simulink model "bike_model"  (R2018a)
settings: Solver=FixedStepAuto  StartTime=0.0  StopTime=10  FixedStep=Ts_IMU  RelTol=1e-3
values from neighbouring files (symbols this model uses):
  A_full = zeros(length(velocity_lqr),3,3)    [bike_init.m]
  A_full_dis = zeros(length(velocity_lqr),3,3)    [bike_init.m]
  amp_dist_roll_rate = 1    [bike_init.m]
  b = 1.095    [bike_init.m]    (also in bike_init_Merged_v1.m = bike3D190215())
  B_full = zeros(length(velocity_lqr),3)    [bike_init.m]
  B_full_dis = zeros(length(velocity_lqr),3)    [bike_init.m]
  C = eye(3)    [bike_init.m]    (also in bike_init_Merged_v1.m)
  complementary = 0.995    [bike_init.m]    (also in bike_init_Merged_v1.m = 0.985)
  cumulative_dist_along_path = [0;cumsum(dist_from_vertex_to_vertex,1)]    [bike_init.m]    (also in bike_init_Merged_v1.m)
  Dead_Band = [0.055,-0.005,0.005]    [bike_init.m]    (also in bike_init_Merged_v1.m = [0.055,-0.055,0.005])
  delay = 0.045    [bike_init.m]    (also in bike_init_Merged_v1.m)
  discrete = 1    [bike_init.m]
  dist_freq = 100    [bike_init.m]
  g = 9.81    [bike_init.m]    (also in bike_init_Merged_v1.m)
  IMU_height = 0.9    [bike_init.m]
  initial_x = x_ini_diff    (= 0)    [bike_init.m]    (also in bike_init_Merged_v1.m)
  initial_y = y_ini_diff    (= 0)    [bike_init.m]    (also in bike_init_Merged_v1.m)
  input_velocity = 2    [bike_init.m]    (also in bike_init_Merged_v1.m = 2.5)
  K_full = zeros(length(velocity_lqr),3)    [bike_init.m]
  K_full_dis = zeros(length(velocity_lqr),3)    [bike_init.m]    (also in bike_init_Merged_v1.m)
  L_full = zeros(length(velocity_lqr),3,3)    [bike_init.m]
  L_full_dis = zeros(length(velocity_lqr),3,3)    [bike_init.m]
  max_handlebar = 40*(pi/180)    (= 0.698131700798)    [bike_init.m]    (also in bike_init_Merged_v1.m)
  max_steering_motor_acc = inf    [bike_init.m]    (also in bike_init_Merged_v1.m)
  max_steering_motor_speed = 7.5    [bike_init.m]    (also in bike_init_Merged_v1.m)
  min_handlebar = -max_handlebar    (= -0.698131700798)    [bike_init.m]    (also in bike_init_Merged_v1.m)
  min_steering_motor_acc = -inf    [bike_init.m]    (also in bike_init_Merged_v1.m)
  min_steering_motor_speed = -7.5    [bike_init.m]    (also in bike_init_Merged_v1.m)
  noise_acc = 0.006*(pi/180)    (= 0.00010471975512)    [bike_init.m]    (also in bike_init_Merged_v1.m)
  noise_encoder = 1e-7    (= 1e-07)    [bike_init.m]    (also in bike_init_Merged_v1.m)
  noise_gyro = 0.001929307*(pi/180)    (= 3.36727594318e-05)    [bike_init.m]    (also in bike_init_Merged_v1.m)
  noise_hall = 0    [bike_init.m]    (also in bike_init_Merged_v1.m)
  parameters = [g h b a]    [bike_init.m]
  path_x = time_array    [bike_init.m]    (also in bike_init_Merged_v1.m)
  path_y = sqrt(path_x * 0.8) .* sin(0.1*path_x)    [bike_init.m]    (also in bike_init_Merged_v1.m)
  roll_rate_coef = 0.8    [bike_init.m]    (also in bike_init_Merged_v1.m = 0.9)
  Ts = 0.04    [bike_init.m]    (also in bike_init_Merged_v1.m)
  Ts_IMU = 0.01    [bike_init.m]    (also in bike_init_Merged_v1.m = 0.04)
  velocity_lqr = linspace(0.001,10,100)    [bike_init.m]    (also in bike_init_Merged_v1.m = [velocity_lqr-0.1 velocity_lqr velocity_lqr+0.1])
undefined symbols (not defined in the file or in its folder): curvature
libraries: simulink x14, dspsigops x2, dspsigattribs x1
(part 1 of 3)
settings Model: Creator=Boaz Ash  LastModifiedBy=Umur

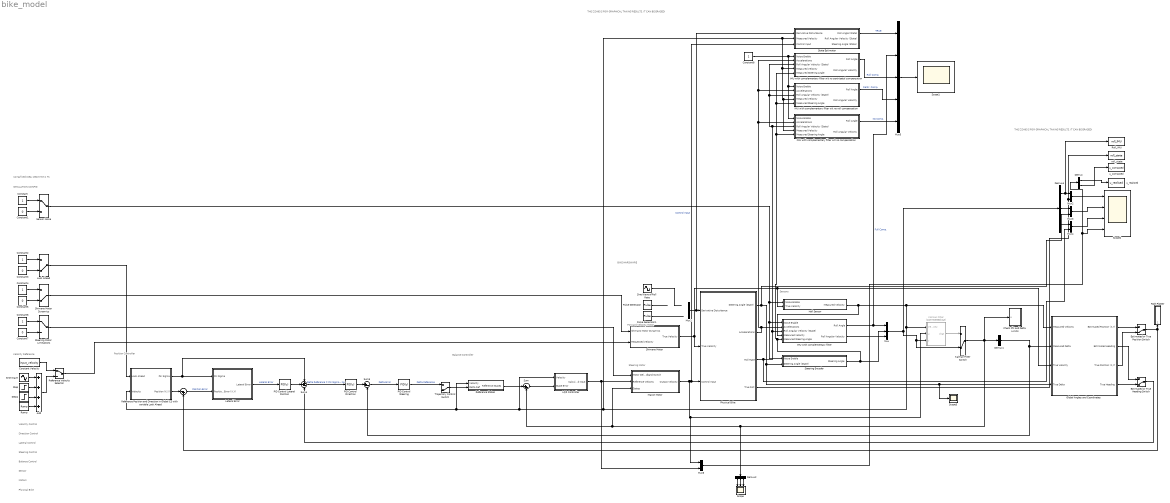
== system bike_model ==
  note: Using fixed step, step time = Ts
  note: SIMULATION CONFIG
  note: BIKE HARDWARE
  note: Direction Control
  note: Steering Control
  note: Lateral Control
  note: Velocity Control
  note: Sensor
  note: Velocity Reference
  note: Sensors
  note: Steering Motor
  note: Balance Control
  note: Forward Velocity Motor
  note: Position Controller
  note: Balance Controller
  note: Motors
  note: Physical Bike
  note: THIS ZONE IS FOR GRAPHICAL TAKING RESULTS. IT CAN BE ERASED!
  note: THIS ZONE IS FOR GRAPHICAL TAKING RESULTS. IT CAN BE ERASED!
  " " : Sum  Inputs=|-+
  Add : Sum  Inputs=4
  Check Phi and Delta Limits : Subsystem  TreatAsAtomicUnit=on  SystemSampleTime=Ts
  Constant{,2,4,6,8} (5 alike) : Constant
  Constant Velocity : Constant  Value=input_velocity
  Constant{1,3,5,7} (4 alike) : Constant  Value=0
  Demux : Demux  Outputs=2
  Demux1 : Demux  Outputs=3
  Demux2 : Demux  Outputs=3
  Demux4 : Demux  Outputs=3
  Estimated or True Heading Switch : ManualSwitch  CurrentSetting=0
  Estimated or True Position Switch : ManualSwitch  CurrentSetting=0
  Global Angles and Coordinates : Subsystem  SystemSampleTime=Ts
  Hall Sensor : Subsystem  TreatAsAtomicUnit=on  SystemSampleTime=Ts
  IMU with complementary filter : Subsystem  SystemSampleTime=Ts_IMU
  IMU with complementary filter wit no centripetal compensation : Subsystem  SystemSampleTime=Ts_IMU
  IMU with complementary filter wit no compensation : Subsystem  SystemSampleTime=Ts_IMU
  IMU with complementary filter wit no roll compensation : Subsystem  SystemSampleTime=Ts_IMU
  Kalman Filter : Subsystem  Commented=on  SystemSampleTime=Ts
  Kalman Filter Switch : ManualSwitch  CurrentSetting=0
  LQR Controller : Subsystem  TreatAsAtomicUnit=on  SystemSampleTime=Ts
  Lateral Error : Subsystem  SystemSampleTime=Ts
  Look Ahead : ManualSwitch  CurrentSetting=0
  Maxon Motor : Subsystem
  Mux : Mux  Inputs=3
  Mux1 : Mux  Inputs=3
  Mux{2..4,6} (4 alike) : Mux  Inputs=2
  Mux5 : Mux  Inputs=5
  PID Control Lateral Position : simulink/Continuous/PID Controller  Controller=PID  TimeDomain=Discrete-time  SampleTime=Ts  IntegratorMethod=Forward Euler  FilterMethod=Forward Euler  Form=Parallel  UseFilter=on  ControllerParametersSource=internal  P=.1  I=.01  D=0  N=100  InitialConditionSource=internal  InitialConditionForIntegrator=0  InitialConditionForFilter=0  ExternalReset=none  LimitOutput=off  UpperSaturationLimit=inf  LowerSaturationLimit=-inf  LinearizeAsGain=on  AntiWindupMode=none  Kb=1  TrackingMode=off  Kt=1  PParamMin=[]  PParamMax=[]  IParamMin=[]  IParamMax=[]  DParamMin=[]  DParamMax=[]  NParamMin=[]  NParamMax=[]  KbParamMin=[]  KbParamMax=[]  KtParamMin=[]  KtParamMax=[]  POutMin=[]  POutMax=[]  IOutMin=[]  IOutMax=[]  DOutMin=[]  DOutMax=[]  NOutMin=[]  NOutMax=[]  KbOutMin=[]  KbOutMax=[]  KtOutMin=[]  KtOutMax=[]  IntegratorOutMin=[]  IntegratorOutMax=[]  FilterOutMin=[]  FilterOutMax=[]  SumOutMin=[]  SumOutMax=[]  SumI1OutMin=[]  SumI1OutMax=[]  SumI2OutMin=[]  SumI2OutMax=[]  SumI3OutMin=[]  SumI3OutMax=[]  SumDOutMin=[]  SumDOutMax=[]  SaturationOutMin=[]  SaturationOutMax=[]  IntegratorContinuousStateAttributes=''  IntegratorStateMustResolveToSignalObject=off  IntegratorRTWStateStorageClass=Auto  FilterContinuousStateAttributes=''  FilterStateMustResolveToSignalObject=off  FilterRTWStateStorageClass=Auto  DifferentiatorICPrevScaledInput=0  DifferentiatorOutMin=[]  DifferentiatorOutMax=[]  FilterDiffOutCoefMin=[]  FilterDiffOutCoefMax=[]  SumDenOutMin=[]  SumDenOutMax=[]  SumNumOutMin=[]  SumNumOutMax=[]  ReciprocalOutMin=[]  ReciprocalOutMax=[]  DivideOutMin=[]  DivideOutMax=[]  TunerSelectOption=Transfer Function Based (PID Tuner App)
  PID Control Direction : simulink/Continuous/PID Controller  Controller=PID  TimeDomain=Discrete-time  SampleTime=Ts  IntegratorMethod=Forward Euler  FilterMethod=Forward Euler  Form=Parallel  UseFilter=on  ControllerParametersSource=internal  P=0.8  I=0.4  D=0  N=100  InitialConditionSource=internal  InitialConditionForIntegrator=0  InitialConditionForFilter=0  ExternalReset=none  LimitOutput=off  UpperSaturationLimit=inf  LowerSaturationLimit=-inf  LinearizeAsGain=on  AntiWindupMode=none  Kb=1  TrackingMode=off  Kt=1  PParamMin=[]  PParamMax=[]  IParamMin=[]  IParamMax=[]  DParamMin=[]  DParamMax=[]  NParamMin=[]  NParamMax=[]  KbParamMin=[]  KbParamMax=[]  KtParamMin=[]  KtParamMax=[]  POutMin=[]  POutMax=[]  IOutMin=[]  IOutMax=[]  DOutMin=[]  DOutMax=[]  NOutMin=[]  NOutMax=[]  KbOutMin=[]  KbOutMax=[]  KtOutMin=[]  KtOutMax=[]  IntegratorOutMin=[]  IntegratorOutMax=[]  FilterOutMin=[]  FilterOutMax=[]  SumOutMin=[]  SumOutMax=[]  SumI1OutMin=[]  SumI1OutMax=[]  SumI2OutMin=[]  SumI2OutMax=[]  SumI3OutMin=[]  SumI3OutMax=[]  SumDOutMin=[]  SumDOutMax=[]  SaturationOutMin=[]  SaturationOutMax=[]  IntegratorContinuousStateAttributes=''  IntegratorStateMustResolveToSignalObject=off  IntegratorRTWStateStorageClass=Auto  FilterContinuousStateAttributes=''  FilterStateMustResolveToSignalObject=off  FilterRTWStateStorageClass=Auto  DifferentiatorICPrevScaledInput=0  DifferentiatorOutMin=[]  DifferentiatorOutMax=[]  FilterDiffOutCoefMin=[]  FilterDiffOutCoefMax=[]  SumDenOutMin=[]  SumDenOutMax=[]  SumNumOutMin=[]  SumNumOutMax=[]  ReciprocalOutMin=[]  ReciprocalOutMax=[]  DivideOutMin=[]  DivideOutMax=[]  TunerSelectOption=Transfer Function Based (PID Tuner App)
  PID Control Steering : simulink/Continuous/PID Controller  Controller=PID  TimeDomain=Discrete-time  SampleTime=Ts  IntegratorMethod=Forward Euler  FilterMethod=Forward Euler  Form=Parallel  UseFilter=on  ControllerParametersSource=internal  P=1  I=0.1  D=0  N=100  InitialConditionSource=internal  InitialConditionForIntegrator=0  InitialConditionForFilter=0  ExternalReset=none  LimitOutput=off  UpperSaturationLimit=inf  LowerSaturationLimit=-inf  LinearizeAsGain=on  AntiWindupMode=none  Kb=1  TrackingMode=off  Kt=1  PParamMin=[]  PParamMax=[]  IParamMin=[]  IParamMax=[]  DParamMin=[]  DParamMax=[]  NParamMin=[]  NParamMax=[]  KbParamMin=[]  KbParamMax=[]  KtParamMin=[]  KtParamMax=[]  POutMin=[]  POutMax=[]  IOutMin=[]  IOutMax=[]  DOutMin=[]  DOutMax=[]  NOutMin=[]  NOutMax=[]  KbOutMin=[]  KbOutMax=[]  KtOutMin=[]  KtOutMax=[]  IntegratorOutMin=[]  IntegratorOutMax=[]  FilterOutMin=[]  FilterOutMax=[]  SumOutMin=[]  SumOutMax=[]  SumI1OutMin=[]  SumI1OutMax=[]  SumI2OutMin=[]  SumI2OutMax=[]  SumI3OutMin=[]  SumI3OutMax=[]  SumDOutMin=[]  SumDOutMax=[]  SaturationOutMin=[]  SaturationOutMax=[]  IntegratorContinuousStateAttributes=''  IntegratorStateMustResolveToSignalObject=off  IntegratorRTWStateStorageClass=Auto  FilterContinuousStateAttributes=''  FilterStateMustResolveToSignalObject=off  FilterRTWStateStorageClass=Auto  DifferentiatorICPrevScaledInput=0  DifferentiatorOutMin=[]  DifferentiatorOutMax=[]  FilterDiffOutCoefMin=[]  FilterDiffOutCoefMax=[]  SumDenOutMin=[]  SumDenOutMax=[]  SumNumOutMin=[]  SumNumOutMax=[]  ReciprocalOutMin=[]  ReciprocalOutMax=[]  DivideOutMin=[]  DivideOutMax=[]  TunerSelectOption=Transfer Function Based (PID Tuner App)
  Path Plotter : Subsystem  SystemSampleTime=Ts
  Physical Bike : Subsystem
  Pulse Generator : DiscretePulseGenerator  PulseType=Time based  Amplitude=pi/36  Period=100  PhaseDelay=0.1
  Pulse Generator1 : DiscretePulseGenerator  PulseType=Time based  Amplitude=0.5*1.1*(20*pi)/36  Period=100  PhaseDelay=1
  Ramp : simulink/Sources/Ramp  slope=0.03  start=0  InitialOutput=0
  Reference Velocity Selector : ManualSwitch
  Reference Position and Direction in Global CS with variable Look Ahead : Subsystem
  Reference States : Subsystem  SystemSampleTime=Ts
  Roll_IMU : ToWorkspace  VariableName=roll_IMU  SaveFormat=Timeseries  SampleTime=-1
  Scope : Scope  NumInputPorts=3
  Scope1 : Scope
  Scope2 : Scope  NumInputPorts=4
  Scope3 : Scope
  Sensor Noise : ManualSwitch
  Shimano Motor : Subsystem
  Shimano Motor Dynamics : ManualSwitch  CurrentSetting=0
  Sine Wave : Sin  Amplitude=0  SampleTime=0
  Sine Wave of Roll Rate : Sin  Amplitude=amp_dist_roll_rate  Frequency=dist_freq  SampleTime=0
  State Estimator : Subsystem
  Steering Encoder : Subsystem  TreatAsAtomicUnit=on  SystemSampleTime=Ts
  Steering Motor Limitations : ManualSwitch
  Step : Step  Time=20  Before=4  After=8  SampleTime=0
  Step1 : Step  Time=40  After=-1  SampleTime=0
  Sum : Sum  Inputs=|+-
  Sum4 : Sum  Inputs=+--
  Sum5 : Sum  Inputs=|+-
  Trajectory Control Switch : ManualSwitch  CurrentSetting=0
  roll_state : ToWorkspace  VariableName=roll_state  SaveFormat=Timeseries  SampleTime=-1
  u_computed : ToWorkspace  VariableName=u_computed  SaveFormat=Timeseries  SampleTime=-1
  u_realised : ToWorkspace  VariableName=u_realised  SaveFormat=Timeseries  SampleTime=-1
  wires:
  Ramp/1 -> Add/4
  Step/1 -> Add/2
  Add/1 -> Reference Velocity Selector/2
  Sine Wave/1 -> Add/1
  Constant Velocity/1 -> Reference Velocity Selector/1
  Step1/1 -> Add/3
  " "/1 -> Lateral Error/2(Position Error (X,Y))  "Position Error"
  Estimated or True Position Switch/1 -> " "/2, Path Plotter/1(Position)
  Lateral Error/1(Lateral Error) -> PID Control Lateral Position/1  "Lateral Error"
  PID Control Steering/1 -> Trajectory Control Switch/1  "Delta Reference"
  Sum5/1 -> PID Control Steering/1  "Delta Error"
  PID Control Direction/1 -> Sum5/1
  Sum4/1 -> PID Control Direction/1  "Delta Reference = Psi Sigma - Nu"
  Reference Position and Direction in Global CS with variable Look Ahead/2(Position (X,Y)) -> " "/1
  Reference Position and Direction in Global CS with variable Look Ahead/1(Psi Sigma) -> Lateral Error/1(Psi Sigma), Sum4/1
  Estimated or True Heading Switch/1 -> Sum4/3
  Maxon Motor/1(Output Velocity) -> State Estimator/3(Control Input), Physical Bike/3(Control Input), Mux6/1, Kalman Filter/2(u)  "Control Input"
  Sum/1 -> LQR Controller/2(State Error)
  Kalman Filter Switch/1 -> Check Phi and Delta Limits/1(x), Sum/2, Maxon Motor/3(States), Demux2/1, Demux1/1
  Constant/1 -> Sensor Noise/1
  Constant1/1 -> Sensor Noise/2
  Sensor Noise/1 -> Hall Sensor/1(Noise Enable), Steering Encoder/1(Noise Enable), IMU with complementary filter/1(Noise Enable)
  IMU with complementary filter/1(Roll Angle) -> Mux/1, Mux5/2  "Full Comp."
  IMU with complementary filter/2(Roll Angular Velocity) -> Mux/3
  Mux1/1 -> State Estimator/1(Derivative Disturbance), Physical Bike/1(Derivative Disturbance)
  Reference States/1(Reference States) -> Sum/1
  Demux1/2 -> Sum5/2, Global Angles and Coordinates/2(Measured Delta)
  Constant3/1 -> Look Ahead/2
  Constant2/1 -> Look Ahead/1
  Look Ahead/1 -> Reference Position and Direction in Global CS with variable Look Ahead/1(Look Ahead)
  Constant4/1 -> Shimano Motor Dynamics/1
  Constant5/1 -> Shimano Motor Dynamics/2
  Global Angles and Coordinates/1(Estimated Position (X,Y)) -> Estimated or True Position Switch/1
  Global Angles and Coordinates/3(True Position (X,Y)) -> Estimated or True Position Switch/2
  Global Angles and Coordinates/2(Estimated Heading) -> Estimated or True Heading Switch/1
  Global Angles and Coordinates/4(True Heading) -> Estimated or True Heading Switch/2
  Reference Velocity Selector/1 -> Shimano Motor/2(Requested Velocity)
  Demux2/1 -> Scope/1
  Demux2/2 -> Scope/2
  Demux2/3 -> Scope/3
  Steering Motor Limitations/1 -> Maxon Motor/1(Motor Delay & Deadband Switch)
  Constant6/1 -> Steering Motor Limitations/1
  Constant7/1 -> Steering Motor Limitations/2
  Mux/1 -> Kalman Filter/3(y), Kalman Filter Switch/2, Demux4/1
  Kalman Filter/1(xhat) -> Kalman Filter Switch/1
  Shimano Motor/1(True Velocity) -> Hall Sensor/2(True Velocity), Global Angles and Coordinates/3(True Velocity), Physical Bike/2(True Velocity)
  Pulse Generator/1 -> ?
  Shimano Motor Dynamics/1 -> Shimano Motor/1(Shimano Motor Dynamics)
  PID Control Lateral Position/1 -> Sum4/2
  Mux2/1 -> Scope2/1
  Mux3/1 -> Scope2/2
  Mux4/1 -> Scope2/3
  Physical Bike/4(True Roll) -> Mux2/2, roll_state/1
  Physical Bike/1(Steering Angle (State)) -> Mux3/2, Steering Encoder/2(Steering Angle (State)), Scope3/1, Global Angles and Coordinates/4(True Delta)
  Demux4/2 -> Mux3/1
  Demux4/3 -> Mux4/1
  Physical Bike/3(Roll Rate) -> Mux4/2, IMU with complementary filter/3(Roll Angular Velocity (State)), IMU with complementary filter wit no centripetal compensation/3(Roll Angular Velocity (State)), IMU with complementary filter wit no roll compensation/3(Roll Angular Velocity (State)), IMU with complementary filter wit no compensation/3(Roll Angular Velocity (State))
  Trajectory Control Switch/1 -> Reference States/2(Delta Ref)
  Pulse Generator1/1 -> ?
  State Estimator/1(Roll Angle (State)) -> Mux5/1  "TRUE"
  Steering Encoder/1(Steering Angle) -> Mux/2, IMU with complementary filter/5(Measured Steering Angle), IMU with complementary filter wit no compensation/5(Measured Steering Angle), IMU with complementary filter wit no roll compensation/5(Measured Steering Angle), IMU with complementary filter wit no centripetal compensation/5(Measured Steering Angle)
  Mux5/1 -> Scope1/1
  Hall Sensor/1(Measured Velocity) -> IMU with complementary filter/4(Measured Velocity), Kalman Filter/1(Velocity), LQR Controller/1(Velocity), Reference States/1(Velocity), Reference Position and Direction in Global CS with variable Look Ahead/2(Velocity), IMU with complementary filter wit no compensation/4(Measured Velocity), IMU with complementary filter wit no roll compensation/4(Measured Velocity), IMU with complementary filter wit no centripetal compensation/4(Measured Velocity), State Estimator/2(Measured Velocity), Global Angles and Coordinates/1(Measured Velocity)
  Physical Bike/2(Accelerations) -> IMU with complementary filter/2(Accelerations), IMU with complementary filter wit no centripetal compensation/2(Accelerations), IMU with complementary filter wit no roll compensation/2(Accelerations), IMU with complementary filter wit no compensation/2(Accelerations)
  Constant8/1 -> IMU with complementary filter wit no compensation/1(Noise Enable), IMU with complementary filter wit no roll compensation/1(Noise Enable), IMU with complementary filter wit no centripetal compensation/1(Noise Enable)
  IMU with complementary filter wit no centripetal compensation/1(Roll Angle) -> Mux5/3  "Roll Comp."
  IMU with complementary filter wit no roll compensation/1(Roll Angle) -> Mux5/4  "Centr. Comp."
  IMU with complementary filter wit no compensation/1(Roll Angle) -> Mux5/5  "No Comp."
  Sine Wave of Roll Rate/1 -> ?
  LQR Controller/1(Calculated Input) -> Mux6/2, Maxon Motor/2(Reference Velocity)
  Mux6/1 -> Scope2/4, Demux/1
  Demux4/1 -> Roll_IMU/1, Mux2/1
  Demux/2 -> u_computed/1
  Demux/1 -> u_realised/1

== system bike_model/Check Phi and Delta Limits ==
  x : Inport
  Demux : Demux  Outputs=3
  Handlebar Lower Bound : simulink/Model Verification/Check Static  Lower Bound  Description=min_handlebar <= u  min=min_handlebar  min_included=on  enabled=on  stopWhenAssertionFail=on  export=on  icon=graphic
      settings: SourceProductName=Simulink
  Handlebar Upper Bound : simulink/Model Verification/Check Static  Upper Bound  Description=u <= max_handlebar  max=max_handlebar  max_included=on  enabled=on  stopWhenAssertionFail=on  export=on  icon=graphic
      settings: SourceProductName=Simulink  SourceProductBaseCode=SL
  Roll Lower Bound : simulink/Model Verification/Check Static  Lower Bound  Description=min_roll <= u  min=min_roll  min_included=on  enabled=on  stopWhenAssertionFail=on  export=on  icon=graphic
      settings: SourceProductName=Simulink
  Roll Upper Bound : simulink/Model Verification/Check Static  Upper Bound  Description=u <= max_roll  max=max_roll  max_included=on  enabled=on  stopWhenAssertionFail=on  export=on  icon=graphic
      settings: SourceProductName=Simulink  SourceProductBaseCode=SL
  wires:
  Demux/1 -> Roll Lower Bound/1, Roll Upper Bound/1  "Roll Angle"
  ? -> Handlebar Upper Bound/1, Handlebar Lower Bound/1  "Handlebar Angle"
  x/1 -> Demux/1

== system bike_model/Global Angles and Coordinates ==
  Measured Velocity : Inport
  Measured Delta : Inport  Port=2
  True Velocity : Inport  Port=3
  True Delta : Inport  Port=4
  Measured Bike Angles to Global Angles : Subsystem
  Measured Global Angles to Global Coordinates : Subsystem
  Sum : Sum  Inputs=++|
  Sum1 : Sum  Inputs=++|
  True Bike Angles to Global Angles2 : Subsystem
  True Global Angles to Global Coordinates : Subsystem
  Estimated Position (X,Y) : Outport
  Estimated Heading : Outport  Port=2
  True Position (X,Y) : Outport  Port=3
  True Heading : Outport  Port=4
  wires:
  Measured Global Angles to Global Coordinates/1("Position (X, Y)") -> Estimated Position (X,Y)/1
  Measured Velocity/1 -> Measured Global Angles to Global Coordinates/1(Velocity), Measured Bike Angles to Global Angles/1(Velocity)
  Measured Bike Angles to Global Angles/1(psi) -> Sum/2, Measured Global Angles to Global Coordinates/2(Psi)
  True Global Angles to Global Coordinates/1("Position (X, Y)") -> True Position (X,Y)/1
  True Delta/1 -> True Bike Angles to Global Angles2/2(Steering Angle)
  True Velocity/1 -> True Global Angles to Global Coordinates/1(Velocity), True Bike Angles to Global Angles2/1(Velocity)
  Measured Bike Angles to Global Angles/2(beta) -> Measured Global Angles to Global Coordinates/3(Beta), Sum/1
  Measured Delta/1 -> Measured Bike Angles to Global Angles/2(Steering Angle)
  Sum/1 -> Estimated Heading/1
  Sum1/1 -> True Heading/1
  True Bike Angles to Global Angles2/1(psi) -> Sum1/2, True Global Angles to Global Coordinates/2(Psi)
  True Bike Angles to Global Angles2/2(beta) -> Sum1/1, True Global Angles to Global Coordinates/3(Beta)

== system bike_model/Hall Sensor ==
  Noise Enable : Inport
  True Velocity : Inport  Port=2
  Noise on hall sensor : RandomNumber  Variance=noise_hall  Seed=1  SampleTime=Ts
  Saturate Signal : Switch  Criteria=u2 > Threshold
  Sum : Sum  Inputs=++|
  Switch : Switch  Criteria=u2 > Threshold
  Velocity Lower Bound : simulink/Model Verification/Check Static  Lower Bound  Description=0.6 <= u  min=0.6  min_included=on  enabled=on  stopWhenAssertionFail=off  export=on  icon=graphic
      settings: SourceProductName=Simulink
  Zero : Constant  Value=0
  Zero-Order Hold : ZeroOrderHold  SampleTime=Ts
  Measured Velocity : Outport
  wires:
  True Velocity/1 -> Sum/2, Switch/3
  Noise Enable/1 -> Switch/2
  Switch/1 -> Saturate Signal/1, Velocity Lower Bound/1
  Noise on hall sensor/1 -> Sum/1
  Sum/1 -> Switch/1
  Zero/1 -> Saturate Signal/3
  Velocity Lower Bound/1 -> Saturate Signal/2
  Saturate Signal/1 -> Zero-Order Hold/1
  Zero-Order Hold/1 -> Measured Velocity/1

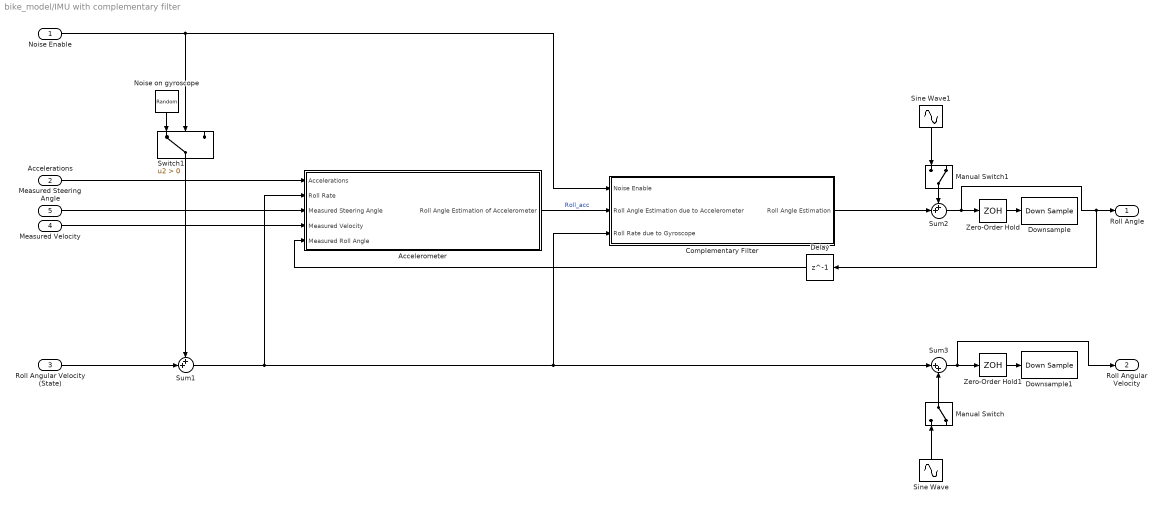
== system bike_model/IMU with complementary filter ==
  Noise Enable : Inport
  Accelerations : Inport  Port=2
  Roll Angular Velocity (State) : Inport  Port=3
  Measured Velocity : Inport  Port=4
  Measured Steering Angle : Inport  Port=5
  Accelerometer : Subsystem
  Complementary Filter : Subsystem  TreatAsAtomicUnit=on  SystemSampleTime=Ts_IMU
  Delay : Delay  DelayLength=1
  Downsample : DownSample  N=Ts/Ts_IMU  RateOptions=Allow multirate processing
  Downsample1 : DownSample  N=Ts/Ts_IMU  RateOptions=Allow multirate processing
  Manual Switch : ManualSwitch  CurrentSetting=0
  Manual Switch1 : ManualSwitch  CurrentSetting=0
  Noise on gyroscope : RandomNumber  Variance=noise_gyro  Seed=1  SampleTime=Ts_IMU
  Sine Wave : Sin  Amplitude=0.05  Frequency=25  SampleTime=Ts_IMU
  Sine Wave1 : Sin  Amplitude=0.02  Frequency=25  Phase=pi  SampleTime=Ts_IMU
  Sum1 : Sum  Inputs=++|
  Sum2 : Sum  Inputs=++|
  Sum3 : Sum  Inputs=|++
  Switch1 : Switch  Criteria=u2 > Threshold
  Zero-Order Hold : ZeroOrderHold  SampleTime=Ts_IMU
  Zero-Order Hold1 : ZeroOrderHold  SampleTime=Ts_IMU
  Roll Angle : Outport
  Roll Angular Velocity : Outport  Port=2
  wires:
  Noise Enable/1 -> Complementary Filter/1(Noise Enable), Switch1/2
  Roll Angular Velocity (State)/1 -> Sum1/2
  Noise on gyroscope/1 -> Switch1/1
  Accelerometer/1(Roll Angle Estimation of Accelerometer) -> Complementary Filter/2(Roll Angle Estimation due to Accelerometer)  "Roll_acc"
  Complementary Filter/1(Roll Angle Estimation) -> Sum2/2
  Switch1/1 -> Sum1/1
  Sine Wave1/1 -> Manual Switch1/1
  Manual Switch1/1 -> Sum2/1
  Sum2/1 -> Delay/1, Roll Angle/1, Zero-Order Hold/1
  Sum3/1 -> Roll Angular Velocity/1, Zero-Order Hold1/1
  Zero-Order Hold/1 -> Downsample/1
  Zero-Order Hold1/1 -> Downsample1/1
  Sum1/1 -> Accelerometer/2(Roll Rate), Complementary Filter/3(Roll Rate due to Gyroscope), Sum3/1
  Sine Wave/1 -> Manual Switch/1
  Manual Switch/1 -> Sum3/2
  Accelerations/1 -> Accelerometer/1(Accelerations)
  Measured Steering Angle/1 -> Accelerometer/3(Measured Steering Angle)
  Measured Velocity/1 -> Accelerometer/4(Measured Velocity)
  Delay/1 -> Accelerometer/5(Measured Roll Angle)

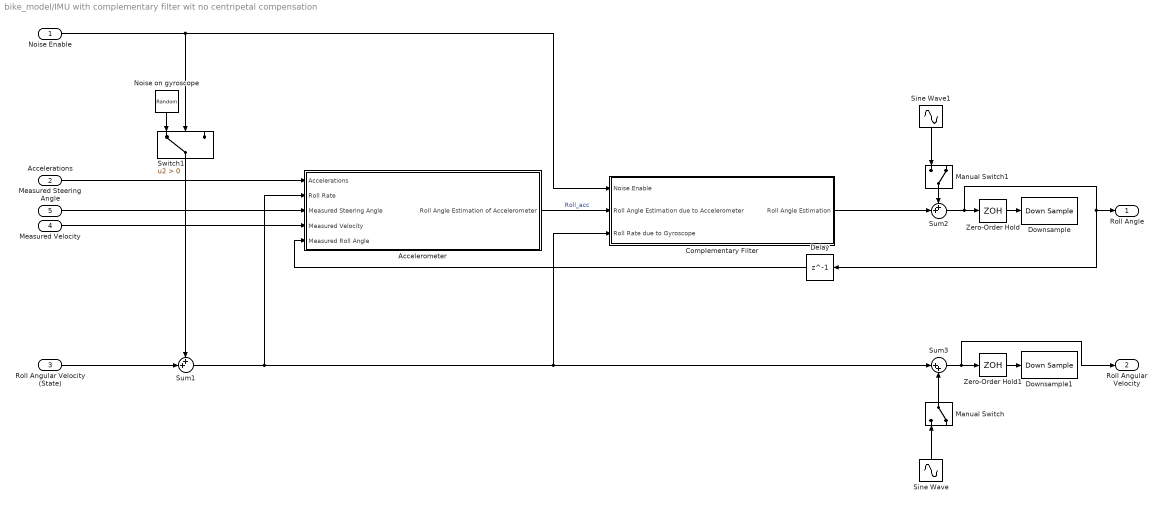
== system bike_model/IMU with complementary filter wit no centripetal compensation ==
  Noise Enable : Inport
  Accelerations : Inport  Port=2
  Roll Angular Velocity (State) : Inport  Port=3
  Measured Velocity : Inport  Port=4
  Measured Steering Angle : Inport  Port=5
  Accelerometer : Subsystem
  Complementary Filter : Subsystem  TreatAsAtomicUnit=on  SystemSampleTime=Ts_IMU
  Delay : Delay  DelayLength=1
  Downsample : DownSample  N=Ts/Ts_IMU  RateOptions=Allow multirate processing
  Downsample1 : DownSample  N=Ts/Ts_IMU  RateOptions=Allow multirate processing
  Manual Switch : ManualSwitch  CurrentSetting=0
  Manual Switch1 : ManualSwitch  CurrentSetting=0
  Noise on gyroscope : RandomNumber  Variance=noise_gyro  Seed=1  SampleTime=Ts_IMU
  Sine Wave : Sin  Amplitude=0.05  Frequency=25  SampleTime=Ts_IMU
  Sine Wave1 : Sin  Amplitude=0.02  Frequency=25  Phase=pi  SampleTime=Ts_IMU
  Sum1 : Sum  Inputs=++|
  Sum2 : Sum  Inputs=++|
  Sum3 : Sum  Inputs=|++
  Switch1 : Switch  Criteria=u2 > Threshold
  Zero-Order Hold : ZeroOrderHold  SampleTime=Ts_IMU
  Zero-Order Hold1 : ZeroOrderHold  SampleTime=Ts_IMU
  Roll Angle : Outport
  Roll Angular Velocity : Outport  Port=2
  wires:
  Noise Enable/1 -> Complementary Filter/1(Noise Enable), Switch1/2
  Roll Angular Velocity (State)/1 -> Sum1/2
  Noise on gyroscope/1 -> Switch1/1
  Accelerometer/1(Roll Angle Estimation of Accelerometer) -> Complementary Filter/2(Roll Angle Estimation due to Accelerometer)  "Roll_acc"
  Complementary Filter/1(Roll Angle Estimation) -> Sum2/2
  Switch1/1 -> Sum1/1
  Sine Wave1/1 -> Manual Switch1/1
  Manual Switch1/1 -> Sum2/1
  Sum2/1 -> Delay/1, Roll Angle/1, Zero-Order Hold/1
  Sum3/1 -> Roll Angular Velocity/1, Zero-Order Hold1/1
  Zero-Order Hold/1 -> Downsample/1
  Zero-Order Hold1/1 -> Downsample1/1
  Sum1/1 -> Accelerometer/2(Roll Rate), Complementary Filter/3(Roll Rate due to Gyroscope), Sum3/1
  Sine Wave/1 -> Manual Switch/1
  Manual Switch/1 -> Sum3/2
  Accelerations/1 -> Accelerometer/1(Accelerations)
  Measured Steering Angle/1 -> Accelerometer/3(Measured Steering Angle)
  Measured Velocity/1 -> Accelerometer/4(Measured Velocity)
  Delay/1 -> Accelerometer/5(Measured Roll Angle)

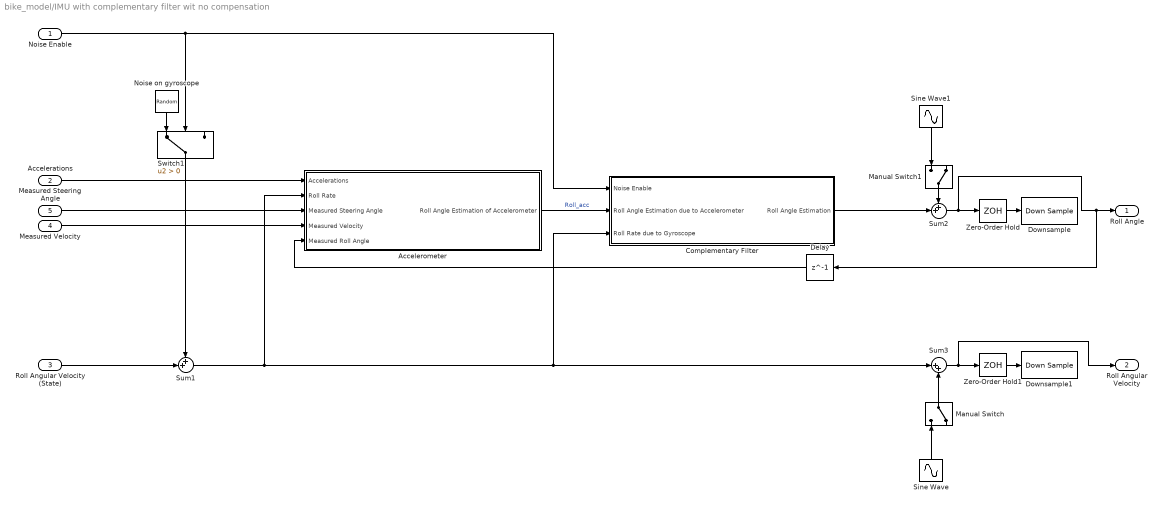
== system bike_model/IMU with complementary filter wit no compensation ==
  Noise Enable : Inport
  Accelerations : Inport  Port=2
  Roll Angular Velocity (State) : Inport  Port=3
  Measured Velocity : Inport  Port=4
  Measured Steering Angle : Inport  Port=5
  Accelerometer : Subsystem
  Complementary Filter : Subsystem  TreatAsAtomicUnit=on  SystemSampleTime=Ts_IMU
  Delay : Delay  DelayLength=1
  Downsample : DownSample  N=Ts/Ts_IMU  RateOptions=Allow multirate processing
  Downsample1 : DownSample  N=Ts/Ts_IMU  RateOptions=Allow multirate processing
  Manual Switch : ManualSwitch  CurrentSetting=0
  Manual Switch1 : ManualSwitch  CurrentSetting=0
  Noise on gyroscope : RandomNumber  Variance=noise_gyro  Seed=1  SampleTime=Ts_IMU
  Sine Wave : Sin  Amplitude=0.05  Frequency=25  SampleTime=Ts_IMU
  Sine Wave1 : Sin  Amplitude=0.02  Frequency=25  Phase=pi  SampleTime=Ts_IMU
  Sum1 : Sum  Inputs=++|
  Sum2 : Sum  Inputs=++|
  Sum3 : Sum  Inputs=|++
  Switch1 : Switch  Criteria=u2 > Threshold
  Zero-Order Hold : ZeroOrderHold  SampleTime=Ts_IMU
  Zero-Order Hold1 : ZeroOrderHold  SampleTime=Ts_IMU
  Roll Angle : Outport
  Roll Angular Velocity : Outport  Port=2
  wires:
  Noise Enable/1 -> Complementary Filter/1(Noise Enable), Switch1/2
  Roll Angular Velocity (State)/1 -> Sum1/2
  Noise on gyroscope/1 -> Switch1/1
  Accelerometer/1(Roll Angle Estimation of Accelerometer) -> Complementary Filter/2(Roll Angle Estimation due to Accelerometer)  "Roll_acc"
  Complementary Filter/1(Roll Angle Estimation) -> Sum2/2
  Switch1/1 -> Sum1/1
  Sine Wave1/1 -> Manual Switch1/1
  Manual Switch1/1 -> Sum2/1
  Sum2/1 -> Delay/1, Roll Angle/1, Zero-Order Hold/1
  Sum3/1 -> Roll Angular Velocity/1, Zero-Order Hold1/1
  Zero-Order Hold/1 -> Downsample/1
  Zero-Order Hold1/1 -> Downsample1/1
  Sum1/1 -> Accelerometer/2(Roll Rate), Complementary Filter/3(Roll Rate due to Gyroscope), Sum3/1
  Sine Wave/1 -> Manual Switch/1
  Manual Switch/1 -> Sum3/2
  Accelerations/1 -> Accelerometer/1(Accelerations)
  Measured Steering Angle/1 -> Accelerometer/3(Measured Steering Angle)
  Measured Velocity/1 -> Accelerometer/4(Measured Velocity)
  Delay/1 -> Accelerometer/5(Measured Roll Angle)

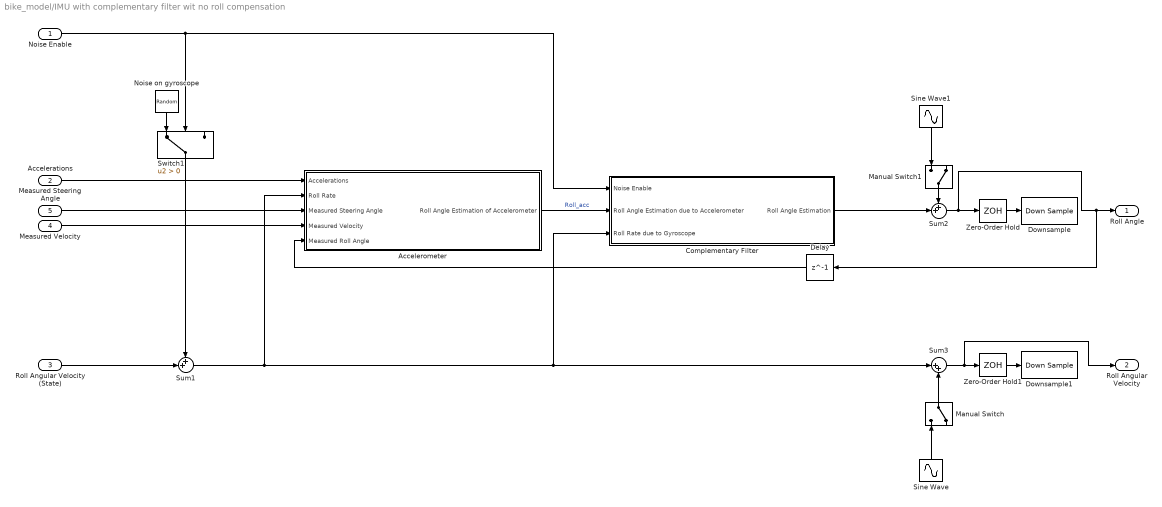
== system bike_model/IMU with complementary filter wit no roll compensation ==
  Noise Enable : Inport
  Accelerations : Inport  Port=2
  Roll Angular Velocity (State) : Inport  Port=3
  Measured Velocity : Inport  Port=4
  Measured Steering Angle : Inport  Port=5
  Accelerometer : Subsystem
  Complementary Filter : Subsystem  TreatAsAtomicUnit=on  SystemSampleTime=Ts_IMU
  Delay : Delay  DelayLength=1
  Downsample : DownSample  N=Ts/Ts_IMU  RateOptions=Allow multirate processing
  Downsample1 : DownSample  N=Ts/Ts_IMU  RateOptions=Allow multirate processing
  Manual Switch : ManualSwitch  CurrentSetting=0
  Manual Switch1 : ManualSwitch  CurrentSetting=0
  Noise on gyroscope : RandomNumber  Variance=noise_gyro  Seed=1  SampleTime=Ts_IMU
  Sine Wave : Sin  Amplitude=0.05  Frequency=25  SampleTime=Ts_IMU
  Sine Wave1 : Sin  Amplitude=0.02  Frequency=25  Phase=pi  SampleTime=Ts_IMU
  Sum1 : Sum  Inputs=++|
  Sum2 : Sum  Inputs=++|
  Sum3 : Sum  Inputs=|++
  Switch1 : Switch  Criteria=u2 > Threshold
  Zero-Order Hold : ZeroOrderHold  SampleTime=Ts_IMU
  Zero-Order Hold1 : ZeroOrderHold  SampleTime=Ts_IMU
  Roll Angle : Outport
  Roll Angular Velocity : Outport  Port=2
  wires:
  Noise Enable/1 -> Complementary Filter/1(Noise Enable), Switch1/2
  Roll Angular Velocity (State)/1 -> Sum1/2
  Noise on gyroscope/1 -> Switch1/1
  Accelerometer/1(Roll Angle Estimation of Accelerometer) -> Complementary Filter/2(Roll Angle Estimation due to Accelerometer)  "Roll_acc"
  Complementary Filter/1(Roll Angle Estimation) -> Sum2/2
  Switch1/1 -> Sum1/1
  Sine Wave1/1 -> Manual Switch1/1
  Manual Switch1/1 -> Sum2/1
  Sum2/1 -> Delay/1, Roll Angle/1, Zero-Order Hold/1
  Sum3/1 -> Roll Angular Velocity/1, Zero-Order Hold1/1
  Zero-Order Hold/1 -> Downsample/1
  Zero-Order Hold1/1 -> Downsample1/1
  Sum1/1 -> Accelerometer/2(Roll Rate), Complementary Filter/3(Roll Rate due to Gyroscope), Sum3/1
  Sine Wave/1 -> Manual Switch/1
  Manual Switch/1 -> Sum3/2
  Accelerations/1 -> Accelerometer/1(Accelerations)
  Measured Steering Angle/1 -> Accelerometer/3(Measured Steering Angle)
  Measured Velocity/1 -> Accelerometer/4(Measured Velocity)
  Delay/1 -> Accelerometer/5(Measured Roll Angle)

== system bike_model/Kalman Filter ==
  Velocity : Inport
  u : Inport  Port=2
  y : Inport  Port=3
  A : Subsystem
  B : Subsystem
  Constant : Constant  Value=discrete
  Convert 1-D to 2-D : dspsigattribs/Convert 1-D to 2-D  M=3  N=1  frameBasedOut=off
      settings: SourceProductName=DSP System Toolbox  SourceProductBaseCode=DS
  Delay : Delay  DelayLength=1  InitialCondition=[0;0;0]
  Gain : Gain  Gain=C  Multiplication=Matrix(K*u)
  Integrator : Integrator
  L : Subsystem
  Product : Product  Multiplication=Matrix(*)
  Product1 : Product  Multiplication=Matrix(*)
  Product4 : Product  Multiplication=Matrix(*)
  Sum : Sum  Inputs=|-+
  Sum1 : Sum  Inputs=+++
  Switch : Switch  Criteria=u2 > Threshold
  xhat : Outport
  wires:
  Gain/1 -> Sum/1
  Sum1/1 -> Delay/1, Integrator/1
  Product/1 -> Sum1/2
  Velocity/1 -> A/1(Velocity), B/1(Velocity), L/1(Velocity)
  u/1 -> Product/2
  y/1 -> Convert 1-D to 2-D/1
  Sum/1 -> Product4/2
  Product4/1 -> Sum1/3
  Switch/1 -> Gain/1, Product1/2, xhat/1
  A/1(A) -> Product1/1
  L/1(L) -> Product4/1
  Product1/1 -> Sum1/1
  Constant/1 -> Switch/2
  Delay/1 -> Switch/1
  Integrator/1 -> Switch/3
  B/1(B) -> Product/1
  Convert 1-D to 2-D/1 -> Sum/2

== system bike_model/LQR Controller ==
  Velocity : Inport
  State Error : Inport  Port=2
  1-D Lookup Table : Lookup_n-D  NumberOfTableDimensions=1  BreakpointsForDimension1=velocity_lqr  BreakpointsForDimension2=velocity_lqr  BreakpointsForDimension3=velocity_lqr  BreakpointsForDimension4=velocity_lqr  Table=K_full_dis(:,1)  InternalRulePriority=Speed  RndMeth=Simplest  InputSameDT=on
  1-D Lookup Table1 : Lookup_n-D  NumberOfTableDimensions=1  BreakpointsForDimension1=velocity_lqr  BreakpointsForDimension2=velocity_lqr  BreakpointsForDimension3=velocity_lqr  BreakpointsForDimension4=velocity_lqr  Table=K_full_dis(:,2)  InternalRulePriority=Speed  RndMeth=Simplest  InputSameDT=on
  1-D Lookup Table2 : Lookup_n-D  NumberOfTableDimensions=1  BreakpointsForDimension1=velocity_lqr  BreakpointsForDimension2=velocity_lqr  BreakpointsForDimension3=velocity_lqr  BreakpointsForDimension4=velocity_lqr  Table=K_full_dis(:,3)  InternalRulePriority=Speed  RndMeth=Simplest  InputSameDT=on
  1-D Lookup Table3 : Lookup_n-D  NumberOfTableDimensions=1  BreakpointsForDimension1=velocity_lqr  BreakpointsForDimension2=velocity_lqr  BreakpointsForDimension3=velocity_lqr  BreakpointsForDimension4=velocity_lqr  Table=K_full(:,1)  InternalRulePriority=Speed  RndMeth=Simplest  InputSameDT=on
  1-D Lookup Table4 : Lookup_n-D  NumberOfTableDimensions=1  BreakpointsForDimension1=velocity_lqr  BreakpointsForDimension2=velocity_lqr  BreakpointsForDimension3=velocity_lqr  BreakpointsForDimension4=velocity_lqr  Table=K_full(:,2)  InternalRulePriority=Speed  RndMeth=Simplest  InputSameDT=on
  1-D Lookup Table5 : Lookup_n-D  NumberOfTableDimensions=1  BreakpointsForDimension1=velocity_lqr  BreakpointsForDimension2=velocity_lqr  BreakpointsForDimension3=velocity_lqr  BreakpointsForDimension4=velocity_lqr  Table=K_full(:,3)  InternalRulePriority=Speed  RndMeth=Simplest  InputSameDT=on
  Constant : Constant  Value=discrete
  Display : Display
  Display1 : Display
  Mux : Mux  Inputs=3
  Mux1 : Mux  Inputs=3
  Product : Product  Multiplication=Matrix(*)
  Switch : Switch  Criteria=u2 > Threshold
  Transpose : Math  Operator=transpose  SaturateOnIntegerOverflow=on
  Zero-Order Hold : ZeroOrderHold  SampleTime=Ts
  Calculated Input : Outport
  wires:
  1-D Lookup Table/1 -> Mux/1  "K1"
  1-D Lookup Table1/1 -> Mux/2  "K2"
  Mux/1 -> Display1/1, Switch/1
  State Error/1 -> Transpose/1
  Product/1 -> Zero-Order Hold/1
  1-D Lookup Table2/1 -> Mux/3  "K3"
  Velocity/1 -> 1-D Lookup Table1/1, 1-D Lookup Table/1, 1-D Lookup Table2/1, 1-D Lookup Table5/1, 1-D Lookup Table4/1, 1-D Lookup Table3/1
  Mux1/1 -> Display/1, Switch/3
  1-D Lookup Table4/1 -> Mux1/2  "K2"
  1-D Lookup Table3/1 -> Mux1/1  "K1"
  1-D Lookup Table5/1 -> Mux1/3  "K3"
  Constant/1 -> Switch/2
  Switch/1 -> Product/2
  Transpose/1 -> Product/1
  Zero-Order Hold/1 -> Calculated Input/1

== system bike_model/Lateral Error ==
  Psi Sigma : Inport
  Position Error (X,Y) : Inport  Port=2
  Cos : Trigonometry  Operator=cos
  Demux : Demux  Outputs=2
  Product : Product
  Product1 : Product
  Sin : Trigonometry
  Sum : Sum  Inputs=+-|
  To Workspace4 : ToWorkspace  VariableName=LAT_ERR  SaveFormat=Timeseries  SampleTime=-1
  Lateral Error : Outport
  wires:
  Cos/1 -> Product/2
  Sin/1 -> Product1/1
  Psi Sigma/1 -> Cos/1, Sin/1
  Product1/1 -> Sum/2
  Product/1 -> Sum/1
  Sum/1 -> To Workspace4/1, Lateral Error/1  "Lateral Error"
  Demux/1 -> Product1/2  "X Position Error"
  Demux/2 -> Product/1  "Y Position Error"
  Position Error (X,Y)/1 -> Demux/1

== system bike_model/Maxon Motor ==
  Motor Delay & Deadband Switch : Inport
  Reference Velocity : Inport  Port=2
  States : Inport  Port=3
  Motor Delay : TransportDelay  DelayTime=delay
  Motor Deadband : Subsystem
  Rate Limiter : RateLimiter  RisingSlewLimit=max_steering_motor_acc  FallingSlewLimit=min_steering_motor_acc  SampleTimeMode=inherited
  Saturation : Saturate  UpperLimit=max_steering_motor_speed  LowerLimit=min_steering_motor_speed
  Switch : Switch  Criteria=u2 > Threshold
  Velocity Saturation wrt Max and Min Handle Bar Angles : Subsystem
  Output Velocity : Outport
  wires:
  Reference Velocity/1 -> Switch/3, Motor Deadband/1(Calculated Input)
  Motor Deadband/1(Input Signal After Dead Band) -> Motor Delay/1
  States/1 -> Velocity Saturation wrt Max and Min Handle Bar Angles/2(States)
  Motor Delay/1 -> Rate Limiter/1
  Motor Delay & Deadband Switch/1 -> Switch/2
  Switch/1 -> Velocity Saturation wrt Max and Min Handle Bar Angles/1(Reference Velocity)
  Rate Limiter/1 -> Saturation/1
  Saturation/1 -> Switch/1
  Velocity Saturation wrt Max and Min Handle Bar Angles/1(Output Velocity) -> Output Velocity/1

== system bike_model/Path Plotter ==
  Position : Inport
  Demux : Demux  Outputs=2
  To Workspace : ToWorkspace  VariableName=X_BIKE  SaveFormat=Timeseries  SampleTime=-1
  To Workspace1 : ToWorkspace  VariableName=Y_BIKE  SaveFormat=Timeseries  SampleTime=-1
  XY Graph : simulink/Sinks/XY Graph  xmin=min(path_x)-5  xmax=max(path_x)+5  ymin=min(path_y)-5  ymax=max(path_y)+5  st=-1
  wires:
  Demux/1 -> XY Graph/1, To Workspace/1  "X"
  Demux/2 -> XY Graph/2, To Workspace1/1  "Y"
  Position/1 -> Demux/1

== system bike_model/Physical Bike ==
  Derivative Disturbance : Inport
  True Velocity : Inport  Port=2
  Control Input : Inport  Port=3
  A (continuous) : Subsystem
  Accelerometer : Subsystem
  B (continuous) : Subsystem
  Centripetal Acceleration Calculator : Subsystem
  Demux : Demux  Outputs=3
  Integrator1 : Integrator  InitialCondition=[0; 0; 0]
  Lateral Acceleration (due to Roll) Calculator : Subsystem
  Matrix Multiply2 : Product  Multiplication=Matrix(*)
  Matrix Multiply3 : Product  Multiplication=Matrix(*)
  Scope : Scope
  Sum1 : Sum  Inputs=+++
  Steering Angle (State) : Outport
  Accelerations : Outport  Port=2
  Roll Rate : Outport  Port=3
  True Roll : Outport  Port=4
  wires:
  Control Input/1 -> Scope/1, Matrix Multiply2/2
  Derivative Disturbance/1 -> Sum1/1
  Matrix Multiply2/1 -> Sum1/2
  Sum1/1 -> Integrator1/1  "X Dot"
  Demux/2 -> Centripetal Acceleration Calculator/1(True Steering Angle), Steering Angle (State)/1  "True Steering Angle"
  Integrator1/1 -> Demux/1, Matrix Multiply3/2  "X"
  Matrix Multiply3/1 -> Sum1/3
  A (continuous)/1(A) -> Matrix Multiply3/1
  B (continuous)/1(B) -> Matrix Multiply2/1
  Centripetal Acceleration Calculator/1(Centripetal Acceleration) -> Accelerometer/2(Centripetal Acceleration due to Path Curvature)
  Lateral Acceleration (due to Roll) Calculator/1(Lateral Acceleration) -> Accelerometer/1(Lateral Acceleration of the IMU due to Roll)
  True Velocity/1 -> Centripetal Acceleration Calculator/2(True Velocity), Accelerometer/3(True Velocity), A (continuous)/1(Velocity), B (continuous)/1(Velocity)
  Accelerometer/1(Accelerations) -> Accelerations/1
  Demux/1 -> True Roll/1, Accelerometer/4(True Roll Angle)  "True Roll Angle"
  Demux/3 -> Roll Rate/1, Lateral Acceleration (due to Roll) Calculator/1(True Roll Rate)  "True Roll Rate"

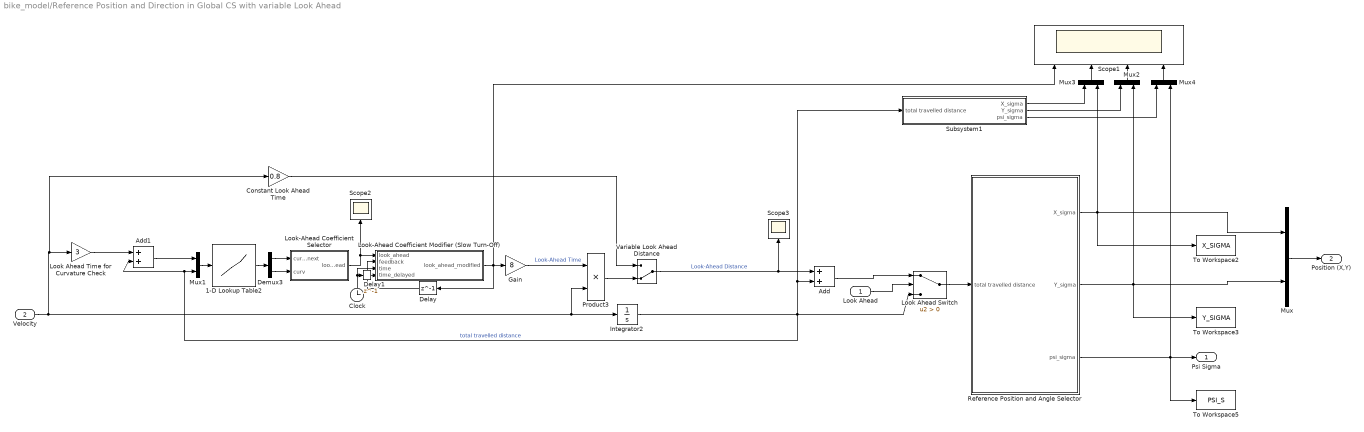
== system bike_model/Reference Position and Direction in Global CS with variable Look Ahead ==
  Look Ahead : Inport
  Velocity : Inport  Port=2
  1-D Lookup Table2 : Lookup_n-D  NumberOfTableDimensions=1  BreakpointsForDimension1=cumulative_dist_along_path  Table=curvature  ExtrapMethod=Clip  DiagnosticForOutOfRangeInput=Error  InternalRulePriority=Speed  RndMeth=Simplest  InputSameDT=on
  Add : Sum
  Add1 : Sum
  Clock : Clock
  Constant Look Ahead Time : Gain  Gain=0.8
  Delay : Delay  DelayLength=1
  Delay1 : Delay  DelayLength=1
  Demux3 : Demux  Outputs=2
  Gain : Gain  Gain=8
  Integrator2 : Integrator
  Look Ahead Switch : Switch  Criteria=u2 > Threshold
  Look Ahead Time for Curvature Check : Gain  Gain=3
  Look-Ahead Coefficient Selector : MATLAB Function  TreatAsAtomicUnit=on
  "Look-Ahead Coefficient Modifier (Slow Turn-Off) " : MATLAB Function  TreatAsAtomicUnit=on
  Mux{,1..4} (5 alike) : Mux  Inputs=2
  Product3 : Product
  Reference Position and Angle Selector : Subsystem
  Scope1 : Scope  NumInputPorts=4
  Scope2 : Scope
  Scope3 : Scope
  Subsystem1 : Subsystem
  To Workspace2 : ToWorkspace  VariableName=X_SIGMA  SaveFormat=Timeseries  SampleTime=-1
  To Workspace3 : ToWorkspace  VariableName=Y_SIGMA  SaveFormat=Timeseries  SampleTime=-1
  To Workspace5 : ToWorkspace  VariableName=PSI_S  SaveFormat=Timeseries  SampleTime=-1
  Variable Look Ahead Distance : ManualSwitch  CurrentSetting=0
  Psi Sigma : Outport
  Position (X,Y) : Outport  Port=2
  wires:
  Constant Look Ahead Time/1 -> Variable Look Ahead Distance/1
  Reference Position and Angle Selector/3(psi_sigma) -> Mux4/2, To Workspace5/1, Psi Sigma/1
  Mux3/1 -> Scope1/2
  Look Ahead Time for Curvature Check/1 -> Add1/1
  Delay/1 -> "Look-Ahead Coefficient Modifier (Slow Turn-Off) "/2(feedback)
  Subsystem1/3(psi_sigma) -> Mux4/1
  Mux2/1 -> Scope1/3
  Clock/1 -> "Look-Ahead Coefficient Modifier (Slow Turn-Off) "/3(time), Delay1/1
  Mux4/1 -> Scope1/4
  Demux3/1 -> Look-Ahead Coefficient Selector/1(curv_next)
  Velocity/1 -> Integrator2/1, Product3/2, Constant Look Ahead Time/1, Look Ahead Time for Curvature Check/1
  Look-Ahead Coefficient Selector/1(look_ahead) -> "Look-Ahead Coefficient Modifier (Slow Turn-Off) "/1(look_ahead), Scope2/1
  Mux1/1 -> 1-D Lookup Table2/1
  "Look-Ahead Coefficient Modifier (Slow Turn-Off) "/1(look_ahead_modified) -> Scope1/1, Delay/1, Gain/1
  1-D Lookup Table2/1 -> Demux3/1
  Demux3/2 -> Look-Ahead Coefficient Selector/2(curv)
  Gain/1 -> Product3/1  "Look-Ahead Time"
  Add/1 -> Look Ahead Switch/1
  Reference Position and Angle Selector/2(Y_sigma) -> Mux/2, Mux2/2, To Workspace3/1
  Look Ahead Switch/1 -> Reference Position and Angle Selector/1(total travelled distance)
  Subsystem1/2(Y_sigma) -> Mux2/1
  Integrator2/1 -> Look Ahead Switch/3, Subsystem1/1(total travelled distance), Add/2, Add1/2, Mux1/2  "total travelled distance"
  Delay1/1 -> "Look-Ahead Coefficient Modifier (Slow Turn-Off) "/4(time_delayed)
  Product3/1 -> Variable Look Ahead Distance/2
  Subsystem1/1(X_sigma) -> Mux3/1
  Reference Position and Angle Selector/1(X_sigma) -> Mux/1, Mux3/2, To Workspace2/1
  Variable Look Ahead Distance/1 -> Scope3/1, Add/1  "Look-Ahead Distance"
  Add1/1 -> Mux1/1
  Look Ahead/1 -> Look Ahead Switch/2
  Mux/1 -> Position (X,Y)/1

== system bike_model/Reference States ==
  Velocity : Inport
  Delta Ref : Inport  Port=2
  Bike Parameters : Constant  Value=parameters
  Mux5 : Mux  Inputs=3
  Reference Roll Angle Calculator : MATLAB Function  TreatAsAtomicUnit=on
  Reference States : Outport
  wires:
  Bike Parameters/1 -> Reference Roll Angle Calculator/1(parameters)
  Delta Ref/1 -> Mux5/2, Reference Roll Angle Calculator/3(delta_ref)
  Reference Roll Angle Calculator/1(phi_ref) -> Mux5/1
  Velocity/1 -> Reference Roll Angle Calculator/2(velocity)
  Mux5/1 -> Reference States/1

== system bike_model/Shimano Motor ==
  note: Add limit for acceleration/deceleration
      | Add min speed of 1.69 m/s (3600 rpm motor speed) limitation
      | Add min speed of 8.20 m/s (18000 rpm motor speed) limitation
      | Add deadband and delay
  Shimano Motor Dynamics : Inport
  Requested Velocity : Inport  Port=2
  Rate Limiter : RateLimiter  RisingSlewLimit=inf  FallingSlewLimit=-inf  SampleTimeMode=inherited
  Saturation : Saturate  UpperLimit=inf  LowerLimit=0
  Switch : Switch  Criteria=u2 > Threshold
  Transfer Fcn : TransferFcn  Numerator=[-0.2156 0.556]  Denominator=[1 1.675 0.5558]
  True Velocity : Outport
  wires:
  Requested Velocity/1 -> Transfer Fcn/1, Switch/3
  Transfer Fcn/1 -> Rate Limiter/1
  Switch/1 -> True Velocity/1
  Shimano Motor Dynamics/1 -> Switch/2
  Saturation/1 -> Switch/1
  Rate Limiter/1 -> Saturation/1

== system bike_model/State Estimator ==
  Derivative Disturbance : Inport
  Measured Velocity : Inport  Port=2
  Control Input : Inport  Port=3
  A (continuous) : Subsystem
  B (continuous) : Subsystem
  Demux : Demux  Outputs=3
  Integrator1 : Integrator  InitialCondition=[0; 0; 0]
  Matrix Multiply2 : Product  Multiplication=Matrix(*)
  Matrix Multiply3 : Product  Multiplication=Matrix(*)
  Scope : Scope
  Sum1 : Sum  Inputs=+++
  Roll Angle (State) : Outport
  Roll Angular Velocity (State) : Outport  Port=2
  Steering Angle (State) : Outport  Port=3
  wires:
  Control Input/1 -> Scope/1, Matrix Multiply2/2
  Derivative Disturbance/1 -> Sum1/1
  Matrix Multiply2/1 -> Sum1/2
  Sum1/1 -> Integrator1/1  "X Dot"
  Demux/2 -> Steering Angle (State)/1
  Demux/1 -> Roll Angle (State)/1
  Demux/3 -> Roll Angular Velocity (State)/1
  Integrator1/1 -> Demux/1, Matrix Multiply3/2  "X"
  Matrix Multiply3/1 -> Sum1/3
  A (continuous)/1(A) -> Matrix Multiply3/1
  Measured Velocity/1 -> A (continuous)/1(Velocity), B (continuous)/1(Velocity)
  B (continuous)/1(B) -> Matrix Multiply2/1

== system bike_model/Steering Encoder ==
  Noise Enable : Inport
  Steering Angle (State) : Inport  Port=2
  Noise on steering encoder : RandomNumber  Variance=noise_encoder  Seed=6  SampleTime=Ts
  Sum : Sum  Inputs=++|
  Switch : Switch  Criteria=u2 > Threshold
  Zero-Order Hold : ZeroOrderHold  SampleTime=Ts
  Steering Angle : Outport
  wires:
  Noise Enable/1 -> Switch/2
  Sum/1 -> Switch/1
  Steering Angle (State)/1 -> Sum/2, Switch/3
  Noise on steering encoder/1 -> Sum/1
  Switch/1 -> Zero-Order Hold/1
  Zero-Order Hold/1 -> Steering Angle/1

== system bike_model/Global Angles and Coordinates/Measured Bike Angles to Global Angles ==
  Velocity : Inport
  Steering Angle : Inport  Port=2
  Integrator : Integrator
  MATLAB Function : MATLAB Function  TreatAsAtomicUnit=on
  Parameters : Constant  Value=parameters
  psi : Outport
  beta : Outport  Port=2
  wires:
  Integrator/1 -> psi/1
  MATLAB Function/1(psi_d) -> Integrator/1
  Steering Angle/1 -> MATLAB Function/3(delta)
  Parameters/1 -> MATLAB Function/2(parameters)
  Velocity/1 -> MATLAB Function/1(v)
  MATLAB Function/2(beta) -> beta/1

== system bike_model/Global Angles and Coordinates/Measured Global Angles to Global Coordinates ==
  Velocity : Inport
  Psi : Inport  Port=2
  Beta : Inport  Port=3
  Constant : Constant  Value=initial_y
  Constant1 : Constant  Value=initial_x
  Integrator1 : Integrator
  Integrator2 : Integrator
  MATLAB Function1 : MATLAB Function  TreatAsAtomicUnit=on
  Mux : Mux  Inputs=2
  Sum : Sum  Inputs=|++
  Sum1 : Sum  Inputs=++|
  "Position (X, Y)" : Outport
  wires:
  MATLAB Function1/2(Ydot) -> Integrator2/1  "Ydot"
  MATLAB Function1/1(Xdot) -> Integrator1/1  "Xdot"
  Psi/1 -> MATLAB Function1/2(psi)
  Beta/1 -> MATLAB Function1/3(beta)
  Velocity/1 -> MATLAB Function1/1(v)
  Integrator2/1 -> Sum/1
  Constant/1 -> Sum/2
  Sum/1 -> Mux/2
  Integrator1/1 -> Sum1/2
  Sum1/1 -> Mux/1
  Constant1/1 -> Sum1/1
  Mux/1 -> "Position (X, Y)"/1

== system bike_model/Global Angles and Coordinates/True Bike Angles to Global Angles2 ==
  Velocity : Inport
  Steering Angle : Inport  Port=2
  Integrator : Integrator
  MATLAB Function : MATLAB Function  TreatAsAtomicUnit=on
  Parameters : Constant  Value=parameters
  To Workspace6 : ToWorkspace  VariableName=PSI  SaveFormat=Timeseries  SampleTime=-1
  To Workspace7 : ToWorkspace  VariableName=BETA  SaveFormat=Timeseries  SampleTime=-1
  psi : Outport
  beta : Outport  Port=2
  wires:
  Integrator/1 -> To Workspace6/1, psi/1
  MATLAB Function/1(psi_d) -> Integrator/1
  Steering Angle/1 -> MATLAB Function/3(delta)
  Parameters/1 -> MATLAB Function/2(parameters)
  Velocity/1 -> MATLAB Function/1(v)
  MATLAB Function/2(beta) -> To Workspace7/1, beta/1

== system bike_model/Global Angles and Coordinates/True Global Angles to Global Coordinates ==
  Velocity : Inport
  Psi : Inport  Port=2
  Beta : Inport  Port=3
  Constant : Constant  Value=initial_y
  Constant1 : Constant  Value=initial_x
  Integrator1 : Integrator
  Integrator2 : Integrator
  MATLAB Function1 : MATLAB Function  TreatAsAtomicUnit=on
  Mux : Mux  Inputs=2
  Sum : Sum  Inputs=|++
  Sum1 : Sum  Inputs=++|
  "Position (X, Y)" : Outport
  wires:
  MATLAB Function1/2(Ydot) -> Integrator2/1  "Ydot"
  MATLAB Function1/1(Xdot) -> Integrator1/1  "Xdot"
  Psi/1 -> MATLAB Function1/2(psi)
  Beta/1 -> MATLAB Function1/3(beta)
  Velocity/1 -> MATLAB Function1/1(v)
  Integrator2/1 -> Sum/1
  Constant/1 -> Sum/2
  Sum/1 -> Mux/2
  Integrator1/1 -> Sum1/2
  Sum1/1 -> Mux/1
  Constant1/1 -> Sum1/1
  Mux/1 -> "Position (X, Y)"/1
